simulink model "Ex2part1"  (R2018b)
settings: Solver=VariableStepAuto  StartTime=0.0  StopTime=10.0  RelTol=1e-3
settings Model: Creator=anton  LastModifiedBy=anton

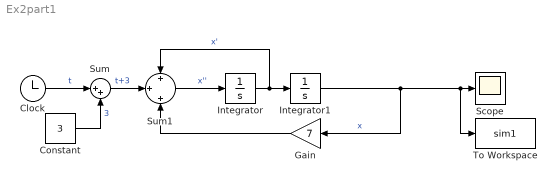
== system Ex2part1 ==
  Clock : Clock
      settings: Decimation=100
  Constant : Constant  Value=3
  Gain : Gain  Gain=7
  Integrator : Integrator  InitialCondition=4
  Integrator1 : Integrator  InitialCondition=3
  Scope : Scope
  Sum : Sum  Inputs=|++
  Sum1 : Sum  Inputs=+|+|+
  To Workspace : ToWorkspace  VariableName=sim1  SaveFormat=Timeseries  SampleTime=-1
  wires:
  Clock/1 -> Sum/1  "t"
  Constant/1 -> Sum/2  "3"
  Sum/1 -> Sum1/2  "t+3"
  Sum1/1 -> Integrator/1  "x''"
  Integrator/1 -> Sum1/1, Integrator1/1  "x'"
  Integrator1/1 -> Scope/1, To Workspace/1, Gain/1  "x"
  Gain/1 -> Sum1/3
